simulink model "NonLinearVehicleiLQR_TP"  (R2020b)
settings: Solver=FixedStepDiscrete  StartTime=0.0  StopTime=50  FixedStep=0.005  MaxStep=0.01  RelTol=1e-3
undefined symbols (not defined in the file): b, DiscIntNeverNeededParam, pos_ref, psi, psi_dot, Q, Qf, R, r, t_ref, vel_ref
libraries: simulink x3
settings Model: Creator=iris  LastModifiedBy=iris

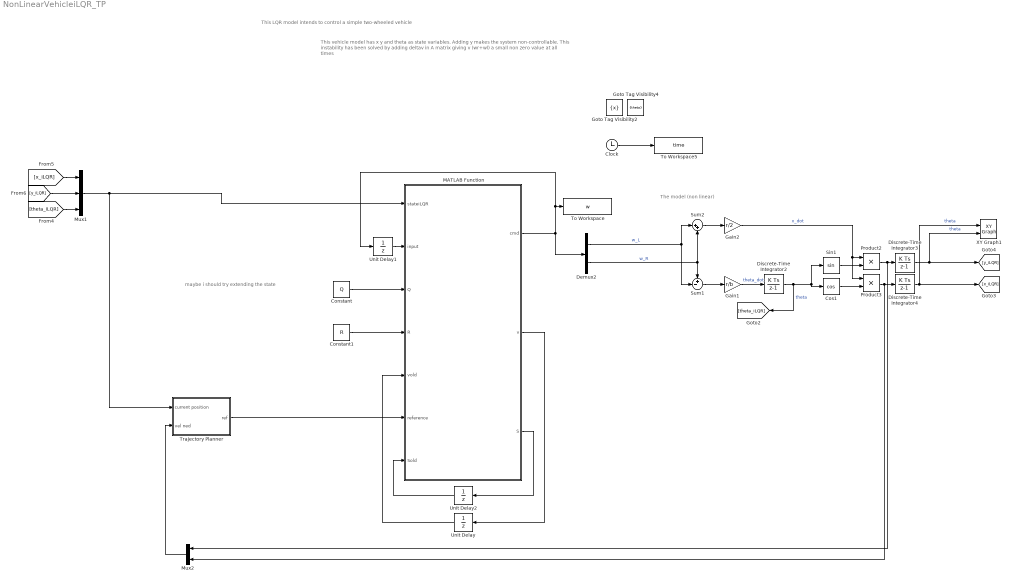
== system NonLinearVehicleiLQR_TP ==
  note: maybe i should try extending the state
  note: The model (non linear)
  note: This vehicle model has x y and theta as state variables. Adding y makes the system non-controllable. This instability has been solved by adding deltav in A matrix giving v (wr+wl) a small non zero value at all times
  note: This LQR model intends to control a simple two-wheeled vehicle
  Clock : Clock
  Constant : Constant  Value=Q
  Constant1 : Constant  Value=R
  Cos1 : Trigonometry  Operator=cos
  Demux2 : Demux  Outputs=2
  Discrete-Time Integrator2 : DiscreteIntegrator  SampleTime=-1  ICPrevOutput=DiscIntNeverNeededParam  ICPrevScaledInput=DiscIntNeverNeededParam
  Discrete-Time Integrator3 : DiscreteIntegrator  SampleTime=-1  ICPrevOutput=DiscIntNeverNeededParam  ICPrevScaledInput=DiscIntNeverNeededParam
  Discrete-Time Integrator4 : DiscreteIntegrator  SampleTime=-1  ICPrevOutput=DiscIntNeverNeededParam  ICPrevScaledInput=DiscIntNeverNeededParam
  Gain1 : Gain  Gain=r/b
  Gain2 : Gain  Gain=r/2
  Goto Tag Visibility2 : GotoTagVisibility  GotoTag=x
  Goto Tag Visibility4 : GotoTagVisibility  GotoTag=theta
  MATLAB Function : MATLAB Function  TreatAsAtomicUnit=on
  Mux1 : Mux  Inputs=3
  Mux2 : Mux  Inputs=2
  Product2 : Product
  Product3 : Product
  Sin1 : Trigonometry
  Sum1 : Sum  Inputs=+-|
  Sum2 : Sum  Inputs=|++
  To Workspace : ToWorkspace  VariableName=w  SampleTime=-1
  To Workspace5 : ToWorkspace  VariableName=time  SampleTime=-1
  Trajectory Planner : Subsystem
  Unit Delay : UnitDelay  InitialCondition=zeros(3,1)  SampleTime=-1  HasFrameUpgradeWarning=on
  Unit Delay1 : UnitDelay  InitialCondition=[0, 0]  SampleTime=-1  HasFrameUpgradeWarning=on
  Unit Delay2 : UnitDelay  InitialCondition=Qf  SampleTime=-1  HasFrameUpgradeWarning=on
  XY Graph1 : simulink/Sinks/XY Graph  xmin=-2  xmax=2  ymin=-2  ymax=2  st=-1
  wires:
  MATLAB Function/3(S) -> Unit Delay2/1
  Unit Delay2/1 -> MATLAB Function/7(Sold)
  MATLAB Function/2(v) -> Unit Delay/1
  Unit Delay/1 -> MATLAB Function/5(vold)
  MATLAB Function/1(cmd) -> Unit Delay1/1, To Workspace/1, Demux2/1
  Constant/1 -> MATLAB Function/3(Q)
  Constant1/1 -> MATLAB Function/4(R)
  Clock/1 -> To Workspace5/1
  Unit Delay1/1 -> MATLAB Function/2(input)
  Gain1/1 -> Discrete-Time Integrator2/1  "theta_dot"
  Sum1/1 -> Gain1/1
  Demux2/1 -> Sum2/1, Sum1/2  "w_L"
  Demux2/2 -> Sum2/2, Sum1/1  "w_R"
  Sum2/1 -> Gain2/1
  Mux1/1 -> Trajectory Planner/1(current position), MATLAB Function/1(stateiLQR)
  [x_iLQR] -> Mux1/1
  [theta_iLQR] -> Mux1/3
  Gain2/1 -> Product3/1, Product2/1  "x_dot"
  Product3/1 -> Mux2/2, Discrete-Time Integrator4/1
  Sin1/1 -> Product2/2
  Discrete-Time Integrator2/1 -> Sin1/1, Cos1/1, [theta_iLQR]  "theta"
  Cos1/1 -> Product3/2
  Product2/1 -> Mux2/1, Discrete-Time Integrator3/1
  [y_iLQR] -> Mux1/2
  Discrete-Time Integrator3/1 -> XY Graph1/2, [y_iLQR]  "theta"
  Discrete-Time Integrator4/1 -> XY Graph1/1, [x_iLQR]  "theta"
  Trajectory Planner/1(ref) -> MATLAB Function/6(reference)
  Mux2/1 -> Trajectory Planner/2(vel ned)

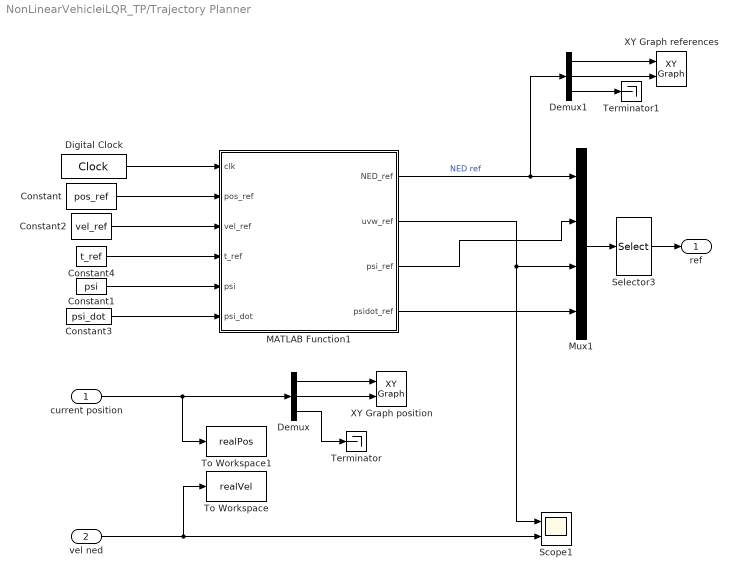
== system NonLinearVehicleiLQR_TP/Trajectory Planner ==
  current position : Inport
  vel ned : Inport  Port=2
  Constant : Constant  Value=pos_ref
  Constant1 : Constant  Value=psi
  Constant2 : Constant  Value=vel_ref
  Constant3 : Constant  Value=psi_dot
  Constant4 : Constant  Value=t_ref
  Demux : Demux  Outputs=3
  Demux1 : Demux  Outputs=3
  Digital Clock : DigitalClock  SampleTime=-1
  MATLAB Function1 : MATLAB Function  TreatAsAtomicUnit=on
  Mux1 : Mux
  Scope1 : Scope  NumInputPorts=2
  Selector3 : Selector  InputPortWidth=8  IndexOptions=Index vector (dialog)  Indices=[1 5 2 6 4 3 7 8]  OutputSizes=1
  Terminator : Terminator
  Terminator1 : Terminator
  To Workspace : ToWorkspace  VariableName=realVel  SaveFormat=Timeseries  SampleTime=-1
  To Workspace1 : ToWorkspace  VariableName=realPos  SaveFormat=Timeseries  SampleTime=-1
  XY Graph position : simulink/Sinks/XY Graph  xmin=-20  xmax=20  ymin=-20  ymax=20  st=-1
  XY Graph references : simulink/Sinks/XY Graph  xmin=-20  xmax=20  ymin=-20  ymax=20  st=-1
  ref : Outport  VectorParamsAs1DForOutWhenUnconnected=off
  wires:
  MATLAB Function1/2(uvw_ref) -> Scope1/1, Mux1/3
  MATLAB Function1/3(psi_ref) -> Mux1/2
  Mux1/1 -> Selector3/1
  MATLAB Function1/1(NED_ref) -> Demux1/1, Mux1/1  "NED ref"
  Selector3/1 -> ref/1
  Constant/1 -> MATLAB Function1/2(pos_ref)
  Constant2/1 -> MATLAB Function1/3(vel_ref)
  current position/1 -> Demux/1, To Workspace1/1
  Demux/2 -> XY Graph position/2
  Demux/1 -> XY Graph position/1
  Demux/3 -> Terminator/1
  Demux1/1 -> XY Graph references/1
  Demux1/2 -> XY Graph references/2
  Demux1/3 -> Terminator1/1
  vel ned/1 -> Scope1/2, To Workspace/1
  Constant4/1 -> MATLAB Function1/4(t_ref)
  Digital Clock/1 -> MATLAB Function1/1(clk)
  Constant1/1 -> MATLAB Function1/5(psi)
  Constant3/1 -> MATLAB Function1/6(psi_dot)
  MATLAB Function1/4(psidot_ref) -> Mux1/4

== matlab function NonLinearVehicleiLQR_TP/MATLAB Function ==
  data: stateiLQR input; cmd output; input input; Q input; R input; vold input; reference input; Sold input; v output; S output
function [cmd, v, S]= fcn(stateiLQR, input , Q, R, vold, reference, Sold)

r = 0.02;
b = 0.185;
dt = 0.001;

% toll = 3*10^-5;

% A = [1 0 dt*-sin(psi)*r/2*(wR+wL);...
%      0 1 dt*cos(psi)*r/2*(wR+wL);...
%      0 0 1];
% B = dt*[cos(psi)*r/2 cos(psi)*r/2;...
%      sin(psi)*r/2 sin(psi)*r/2;...
%      -r/b r/b];
% A = eye(3);
% B = dt*[r/2 r/2;
%      0 0;
%      -r/b r/b];
deltav = 0.00001; % this ensures the system is controllable everytime
% A = [1 0 dt*-sin(psi)*r/2*(wR+wL+deltav);...
%      0 1 dt*cos(psi)*r/2*(wR+wL+deltav);...
%      0 0 1];
% B = dt*[cos(psi)*r/2 cos(psi)*r/2;...
%      sin(psi)*r/2 sin(psi)*r/2;...
%      -r/b r/b];
% A = [1 dt*r/2*(sum(input));
%     0 1];
% B = dt*[r/2 r/2;
%     -r/b r/b];

state = stateiLQR';
psi = stateiLQR(3);
wR = input(2);
wL = input(1);
A = [1 0 dt*-sin(psi)*r/2*(wR+wL+deltav);...
     0 1 dt*cos(psi)*r/2*(wR+wL+deltav);...
     0 0 1];
B = dt*[cos(psi)*r/2 cos(psi)*r/2;...
     sin(psi)*r/2 sin(psi)*r/2;...
     -r/b r/b];
 
K  = (B'*Sold*B+R)\B'*Sold*A;
Kv = (B'*Sold*B+R)\B';
Ku = (B'*Sold*B+R)\R;
S  = A'*Sold*(A-B*K)+Q;
deltax = [-reference(1);-reference(3);-reference(5)]; % Changed the sign on this one because
% otherwise, the state is mirrored to the reference
v  = (A-B*K)'*vold+Q*deltax-K'*R*input;
deltau = -K*state'-Kv*v-Ku*input;
cmd  = input + deltau;

end

== matlab function NonLinearVehicleiLQR_TP/Trajectory Planner/MATLAB Function1 ==
  data: clk input; NED_ref output; pos_ref input; vel_ref input; t_ref input; uvw_ref output; psi input; psi_ref output; psi_dot input; psidot_ref output
function [ NED_ref, uvw_ref, psi_ref,psidot_ref] = trajectoryPlanner(clk,pos_ref,vel_ref,t_ref,psi,psi_dot)

currTime = find(clk >= t_ref);
NED_ref = pos_ref(currTime(end),:);
uvw_ref = vel_ref(currTime(end),:);
psi_ref = psi(currTime(end),:);
psidot_ref = psi_dot(currTime(end),:);
end
